simulink model "TxLUT_RxCapture_4x4_HDL_IQ"  (R2019b)
settings: Solver=FixedStepDiscrete  StartTime=0.0  StopTime=15e3  RelTol=1e-3
PreLoadFcn:
  | load('iq_bus_obj.mat');
  | model_init
InitFcn:
  | model_init
values from neighbouring files (symbols this model uses):
  FPGAClkRate = DataSampleRate/VectorSamplingFactor    (= 128000000)    [model_init.m]
  RAM_addr_width = nextpow2(RAM_num_entries)    [model_init.m]
  S2MM_frame_size = 5e4    (= 50000)    [host_io_model_init.m]    (also in model_init.m = length(signal))
  signal = exp(2j*pi*(k/2*t+f0).*t)    [model_init.m]
libraries: hdlsllib x26, simulink x14, rfsoc_hdl_utils x5, dspsrcs4 x2
Description:
  | HDL model for RFSoC ADC/DAC IQ 8x8 interfacing with the mixer enabled
  | 
  | This model contains demonstrates how to interface to all 8 ADC and 8 DAC
  | channels for the RFSoC.
  | 
  | Please ensure that you run the initialization script to set the correct PLL clock rates.
settings Model: DataTypeOverride=Off  SimulationMode=accelerator  Creator=mfornero  LastModifiedBy=ajtro
settings DataIOCC: SaveOutput=off  SaveTime=off  ReturnWorkspaceOutputs=off
settings OptimizationCC: BlockReduction=off  ConditionallyExecuteInputs=off  DefaultParameterBehavior=Inlined  LifeSpan=inf
settings DebuggingCC: AlgebraicLoopMsg=error  SingleTaskRateTransMsg=error  PregeneratedLibrarySubsystemCodeDiagnostic=none  StrictBusMsg=ErrorOnBusTreatedAsVector  SFUnexpectedBacktrackingDiag=warning  SFNoUnconditionalDefaultTransitionDiag=warning  SFExecutionAtInitializationDiag=none  ArithmeticOperatorsInVariantConditions=warning
settings HardwareCC: ProdBitPerPointer=32  ProdBitPerSizeT=32  ProdBitPerPtrDiffT=32  ProdLargestAtomicFloat=None  ProdIntDivRoundTo=Undefined  ProdEndianess=Unspecified  ProdWordSize=32  ProdHWDeviceType=ASIC/FPGA->ASIC/FPGA  ProdEqTarget=off
settings SFSimCC: SimUseLocalCustomCode=off  CustomCodeUndefinedFunction=UseInterfaceOnly
settings RTWCC: RTWUseLocalCustomCode=off
settings CodeAppCC: StateflowObjectComments=on
settings GRTTargetCC: TargetLangStandard=C89/C90 (ANSI)
settings ConfigComp: CovMetricSettings=dw  CovHtmlReporting=on  CovSaveCumulativeToWorkspaceVar=on  CovSaveSingleToWorkspaceVar=on  CovExternalEMLEnable=off

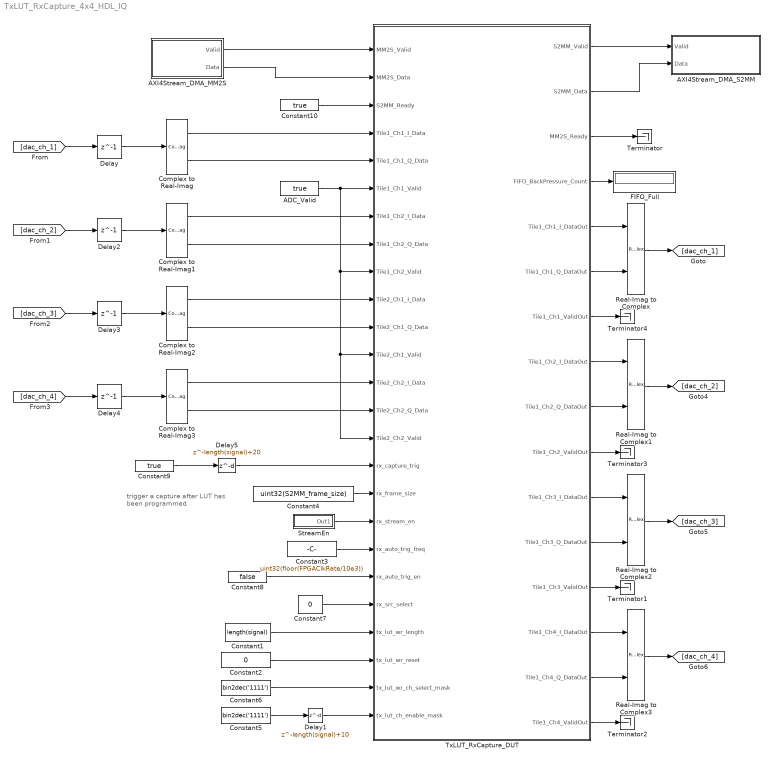
== system TxLUT_RxCapture_4x4_HDL_IQ ==
  note: trigger a capture after LUT
      | has been programmed
  ADC_Valid : Constant  Value=true  SampleTime=-1
  AXI4Stream_DMA_MM2S : Subsystem
  AXI4Stream_DMA_S2MM : Subsystem
  Complex to Real-Imag{,1..3} (4 alike) : ComplexToRealImag
  Constant1 : Constant  Value=length(signal)  OutDataTypeStr=uint32  SampleTime=-1
  Constant10 : Constant  Value=true  SampleTime=-1
  Constant2 : Constant  Value=0  OutDataTypeStr=boolean  SampleTime=-1
  Constant3 : Constant  Value=uint32(floor(FPGAClkRate/10e3))  OutDataTypeStr=uint32  SampleTime=-1
  Constant4 : Constant  Value=uint32(S2MM_frame_size)  SampleTime=-1
  Constant5 : Constant  Value=bin2dec('1111')  OutDataTypeStr=uint32  SampleTime=-1
  Constant6 : Constant  Value=bin2dec('1111')  OutDataTypeStr=uint32  SampleTime=-1
  Constant7 : Constant  Value=0  OutDataTypeStr=fixdt(0,1,0)  SampleTime=-1
  Constant8 : Constant  Value=false  SampleTime=-1
  Constant9 : Constant  Value=true  SampleTime=-1
  Delay{,2..4} (4 alike) : Delay  DelayLength=1
  Delay1 : Delay  DelayLength=length(signal)+10
  Delay5 : Delay  DelayLength=length(signal)+20
  FIFO_Full : Display
  Real-Imag to Complex{,1..3} (4 alike) : RealImagToComplex
  StreamEn : Subsystem
  Terminator{,1..4} (5 alike) : Terminator
  TxLUT_RxCapture_DUT : Subsystem  TreatAsAtomicUnit=on
  wires:
  Constant4/1 -> TxLUT_RxCapture_DUT/17(rx_frame_size)
  StreamEn/1(Out1) -> TxLUT_RxCapture_DUT/18(rx_stream_en)
  Constant3/1 -> TxLUT_RxCapture_DUT/19(rx_auto_trig_freq)
  TxLUT_RxCapture_DUT/1(S2MM_Valid) -> AXI4Stream_DMA_S2MM/1(Valid)
  TxLUT_RxCapture_DUT/2(S2MM_Data) -> AXI4Stream_DMA_S2MM/2(Data)
  TxLUT_RxCapture_DUT/3(MM2S_Ready) -> Terminator/1
  ADC_Valid/1 -> TxLUT_RxCapture_DUT/9(Tile1_Ch2_Valid), TxLUT_RxCapture_DUT/12(Tile2_Ch1_Valid), TxLUT_RxCapture_DUT/15(Tile2_Ch2_Valid), TxLUT_RxCapture_DUT/6(Tile1_Ch1_Valid)
  Constant1/1 -> TxLUT_RxCapture_DUT/22(tx_lut_wr_length)
  AXI4Stream_DMA_MM2S/1(Valid) -> TxLUT_RxCapture_DUT/1(MM2S_Valid)
  AXI4Stream_DMA_MM2S/2(Data) -> TxLUT_RxCapture_DUT/2(MM2S_Data)
  Constant10/1 -> TxLUT_RxCapture_DUT/3(S2MM_Ready)
  Constant2/1 -> TxLUT_RxCapture_DUT/23(tx_lut_wr_reset)
  Constant5/1 -> Delay1/1
  Constant6/1 -> TxLUT_RxCapture_DUT/24(tx_lut_wr_ch_select_mask)
  Complex to Real-Imag/1 -> TxLUT_RxCapture_DUT/4("Tile1_Ch1_I_Data ")
  Delay/1 -> Complex to Real-Imag/1
  Delay1/1 -> TxLUT_RxCapture_DUT/25(tx_lut_ch_enable_mask)
  Complex to Real-Imag/2 -> TxLUT_RxCapture_DUT/5(Tile1_Ch1_Q_Data)
  Constant7/1 -> TxLUT_RxCapture_DUT/21(rx_src_select)
  TxLUT_RxCapture_DUT/5(Tile1_Ch1_I_DataOut) -> Real-Imag to Complex/1
  TxLUT_RxCapture_DUT/6(Tile1_Ch1_Q_DataOut) -> Real-Imag to Complex/2
  TxLUT_RxCapture_DUT/4(FIFO_BackPressure_Count) -> FIFO_Full/1
  TxLUT_RxCapture_DUT/8(Tile1_Ch2_I_DataOut) -> Real-Imag to Complex1/1
  TxLUT_RxCapture_DUT/9(Tile1_Ch2_Q_DataOut) -> Real-Imag to Complex1/2
  TxLUT_RxCapture_DUT/11(Tile1_Ch3_I_DataOut) -> Real-Imag to Complex2/1
  TxLUT_RxCapture_DUT/12(Tile1_Ch3_Q_DataOut) -> Real-Imag to Complex2/2
  TxLUT_RxCapture_DUT/14(Tile1_Ch4_I_DataOut) -> Real-Imag to Complex3/1
  TxLUT_RxCapture_DUT/15(Tile1_Ch4_Q_DataOut) -> Real-Imag to Complex3/2
  TxLUT_RxCapture_DUT/13(Tile1_Ch3_ValidOut) -> Terminator1/1
  TxLUT_RxCapture_DUT/16(Tile1_Ch4_ValidOut) -> Terminator2/1
  TxLUT_RxCapture_DUT/10(Tile1_Ch2_ValidOut) -> Terminator3/1
  TxLUT_RxCapture_DUT/7(Tile1_Ch1_ValidOut) -> Terminator4/1
  Real-Imag to Complex/1 -> [dac_ch_1]
  Real-Imag to Complex1/1 -> [dac_ch_2]
  Real-Imag to Complex2/1 -> [dac_ch_3]
  Real-Imag to Complex3/1 -> [dac_ch_4]
  [dac_ch_1] -> Delay/1
  [dac_ch_2] -> Delay2/1
  Complex to Real-Imag1/2 -> TxLUT_RxCapture_DUT/8(Tile1_Ch2_Q_Data)
  Delay2/1 -> Complex to Real-Imag1/1
  Complex to Real-Imag1/1 -> TxLUT_RxCapture_DUT/7(Tile1_Ch2_I_Data)
  Complex to Real-Imag2/1 -> TxLUT_RxCapture_DUT/10(Tile2_Ch1_I_Data)
  Delay3/1 -> Complex to Real-Imag2/1
  Complex to Real-Imag2/2 -> TxLUT_RxCapture_DUT/11(Tile2_Ch1_Q_Data)
  [dac_ch_3] -> Delay3/1
  [dac_ch_4] -> Delay4/1
  Complex to Real-Imag3/2 -> TxLUT_RxCapture_DUT/14(Tile2_Ch2_Q_Data)
  Delay4/1 -> Complex to Real-Imag3/1
  Complex to Real-Imag3/1 -> TxLUT_RxCapture_DUT/13(Tile2_Ch2_I_Data)
  Constant8/1 -> TxLUT_RxCapture_DUT/20(rx_auto_trig_en)
  Constant9/1 -> Delay5/1
  Delay5/1 -> TxLUT_RxCapture_DUT/16(rx_capture_trig)

== system TxLUT_RxCapture_4x4_HDL_IQ/AXI4Stream_DMA_MM2S ==
  note: Simple behavioral model for MM2S DMA
  Data Type Conversion : DataTypeConversion  OutDataTypeStr=fixdt(0,128,0)  ConvertRealWorld=Stored Integer (SI)
  Pack Complex : rfsoc_hdl_utils/Pack Complex  dummy=0
  Signal From Workspace : dspsrcs4/Signal From Workspace  X=signal_int16  Ts=1  nsamps=1  OutputAfterFinalValue=Setting to zero  ignoreOrWarnInputAndFrameLengths=off  OutputFrames=off
  Signal From Workspace1 : dspsrcs4/Signal From Workspace  X=true(length(signal),1)  Ts=1  nsamps=1  OutputAfterFinalValue=Setting to zero  ignoreOrWarnInputAndFrameLengths=off  OutputFrames=off
  Valid : Outport  VectorParamsAs1DForOutWhenUnconnected=off
  Data : Outport  Port=2  VectorParamsAs1DForOutWhenUnconnected=off
  wires:
  Signal From Workspace/1 -> Pack Complex/1
  Signal From Workspace1/1 -> Valid/1
  Data Type Conversion/1 -> Data/1
  Pack Complex/1 -> Data Type Conversion/1

== system TxLUT_RxCapture_4x4_HDL_IQ/AXI4Stream_DMA_S2MM ==
  Valid : Inport
  Data : Inport  Port=2
  PlotData : Subsystem
  wires:
  Valid/1 -> PlotData/Enable
  Data/1 -> PlotData/1(In1)

== system TxLUT_RxCapture_4x4_HDL_IQ/StreamEn ==
  Data Type Conversion1 : DataTypeConversion  OutDataTypeStr=boolean
  Manual Switch1 : ManualSwitch
  OFF : Constant  Value=0  OutDataTypeStr=boolean  SampleTime=-1
  ON : Constant  OutDataTypeStr=boolean  SampleTime=-1
  Out1 : Outport  VectorParamsAs1DForOutWhenUnconnected=off
  wires:
  Data Type Conversion1/1 -> Out1/1
  OFF/1 -> Manual Switch1/2
  ON/1 -> Manual Switch1/1
  Manual Switch1/1 -> Data Type Conversion1/1

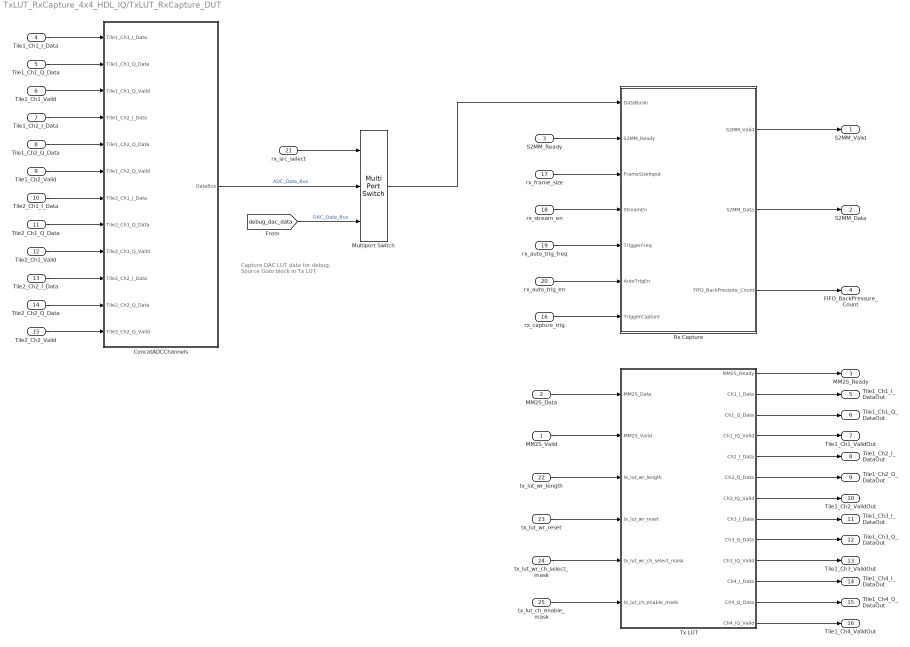
== system TxLUT_RxCapture_4x4_HDL_IQ/TxLUT_RxCapture_DUT ==
  note: Capture DAC LUT data for debug,
      | Source Goto block in Tx LUT
  MM2S_Valid : Inport
  MM2S_Data : Inport  Port=2
  S2MM_Ready : Inport  Port=3
  "Tile1_Ch1_I_Data " : Inport  Port=4
  Tile1_Ch1_Q_Data : Inport  Port=5
  Tile1_Ch1_Valid : Inport  Port=6
  Tile1_Ch2_I_Data : Inport  Port=7
  Tile1_Ch2_Q_Data : Inport  Port=8
  Tile1_Ch2_Valid : Inport  Port=9
  Tile2_Ch1_I_Data : Inport  Port=10
  Tile2_Ch1_Q_Data : Inport  Port=11
  Tile2_Ch1_Valid : Inport  Port=12
  Tile2_Ch2_I_Data : Inport  Port=13
  Tile2_Ch2_Q_Data : Inport  Port=14
  Tile2_Ch2_Valid : Inport  Port=15
  rx_capture_trig : Inport  Port=16
  rx_frame_size : Inport  Port=17
  rx_stream_en : Inport  Port=18
  rx_auto_trig_freq : Inport  Port=19
  rx_auto_trig_en : Inport  Port=20
  rx_src_select : Inport  Port=21  OutDataTypeStr=fixdt(0,1,0)
  tx_lut_wr_length : Inport  Port=22
  tx_lut_wr_reset : Inport  Port=23
  tx_lut_wr_ch_select_mask : Inport  Port=24
  tx_lut_ch_enable_mask : Inport  Port=25
  ConcatADCChannels : Subsystem
  Multiport Switch : MultiPortSwitch  DataPortOrder=Zero-based contiguous  Inputs=2  zeroidx=on
  Rx Capture : Subsystem
  Tx LUT : Subsystem
  S2MM_Valid : Outport  VectorParamsAs1DForOutWhenUnconnected=off
  S2MM_Data : Outport  Port=2  VectorParamsAs1DForOutWhenUnconnected=off
  MM2S_Ready : Outport  Port=3  VectorParamsAs1DForOutWhenUnconnected=off
  FIFO_BackPressure_Count : Outport  Port=4  VectorParamsAs1DForOutWhenUnconnected=off
  Tile1_Ch1_I_DataOut : Outport  Port=5  VectorParamsAs1DForOutWhenUnconnected=off
  Tile1_Ch1_Q_DataOut : Outport  Port=6  VectorParamsAs1DForOutWhenUnconnected=off
  Tile1_Ch1_ValidOut : Outport  Port=7  VectorParamsAs1DForOutWhenUnconnected=off
  Tile1_Ch2_I_DataOut : Outport  Port=8  VectorParamsAs1DForOutWhenUnconnected=off
  Tile1_Ch2_Q_DataOut : Outport  Port=9  VectorParamsAs1DForOutWhenUnconnected=off
  Tile1_Ch2_ValidOut : Outport  Port=10  VectorParamsAs1DForOutWhenUnconnected=off
  Tile1_Ch3_I_DataOut : Outport  Port=11  VectorParamsAs1DForOutWhenUnconnected=off
  Tile1_Ch3_Q_DataOut : Outport  Port=12  VectorParamsAs1DForOutWhenUnconnected=off
  Tile1_Ch3_ValidOut : Outport  Port=13  VectorParamsAs1DForOutWhenUnconnected=off
  Tile1_Ch4_I_DataOut : Outport  Port=14  VectorParamsAs1DForOutWhenUnconnected=off
  Tile1_Ch4_Q_DataOut : Outport  Port=15  VectorParamsAs1DForOutWhenUnconnected=off
  Tile1_Ch4_ValidOut : Outport  Port=16  VectorParamsAs1DForOutWhenUnconnected=off
  wires:
  Tx LUT/1(MM2S_Ready) -> MM2S_Ready/1
  S2MM_Ready/1 -> Rx Capture/2(S2MM_Ready)
  rx_frame_size/1 -> Rx Capture/3(FrameSizeInput)
  rx_stream_en/1 -> Rx Capture/4(StreamEn)
  rx_auto_trig_freq/1 -> Rx Capture/5(TriggerFreq)
  rx_auto_trig_en/1 -> Rx Capture/6(AutoTrigEn)
  rx_capture_trig/1 -> Rx Capture/7(TriggerCapture)
  Rx Capture/1(S2MM_Valid) -> S2MM_Valid/1
  Rx Capture/2(S2MM_Data) -> S2MM_Data/1
  Rx Capture/3(FIFO_BackPressure_Count) -> FIFO_BackPressure_Count/1
  MM2S_Data/1 -> Tx LUT/1(MM2S_Data)
  MM2S_Valid/1 -> Tx LUT/2(MM2S_Valid)
  tx_lut_wr_ch_select_mask/1 -> Tx LUT/5(tx_lut_wr_ch_select_mask)
  tx_lut_wr_length/1 -> Tx LUT/3(tx_lut_wr_length)
  tx_lut_wr_reset/1 -> Tx LUT/4(tx_lut_wr_reset)
  tx_lut_ch_enable_mask/1 -> Tx LUT/6(tx_lut_ch_enable_mask)
  "Tile1_Ch1_I_Data "/1 -> ConcatADCChannels/1("Tile1_Ch1_I_Data ")
  Tile1_Ch1_Q_Data/1 -> ConcatADCChannels/2(Tile1_Ch1_Q_Data)
  Tile1_Ch1_Valid/1 -> ConcatADCChannels/3(Tile1_Ch1_Q_Valid)
  Tile1_Ch2_I_Data/1 -> ConcatADCChannels/4(Tile1_Ch2_I_Data)
  Tile1_Ch2_Q_Data/1 -> ConcatADCChannels/5(Tile1_Ch2_Q_Data)
  Tile1_Ch2_Valid/1 -> ConcatADCChannels/6(Tile1_Ch2_Q_Valid)
  Tile2_Ch1_I_Data/1 -> ConcatADCChannels/7(Tile2_Ch1_I_Data)
  Tile2_Ch1_Q_Data/1 -> ConcatADCChannels/8(Tile2_Ch1_Q_Data)
  Tile2_Ch1_Valid/1 -> ConcatADCChannels/9(Tile2_Ch1_Q_Valid)
  Tile2_Ch2_I_Data/1 -> ConcatADCChannels/10(Tile2_Ch2_I_Data)
  Tile2_Ch2_Q_Data/1 -> ConcatADCChannels/11(Tile2_Ch2_Q_Data)
  Tile2_Ch2_Valid/1 -> ConcatADCChannels/12(Tile2_Ch2_Q_Valid)
  [debug_dac_data] -> Multiport Switch/3  "DAC_Data_Bus"
  ConcatADCChannels/1(DataBus) -> Multiport Switch/2  "ADC_Data_Bus"
  Multiport Switch/1 -> Rx Capture/1(DataBusIn)
  rx_src_select/1 -> Multiport Switch/1
  Tx LUT/2(Ch1_I_Data) -> Tile1_Ch1_I_DataOut/1
  Tx LUT/11(Ch4_I_Data) -> Tile1_Ch4_I_DataOut/1
  Tx LUT/10(Ch3_IQ_Valid) -> Tile1_Ch3_ValidOut/1
  Tx LUT/13(Ch4_IQ_Valid) -> Tile1_Ch4_ValidOut/1
  Tx LUT/5(Ch2_I_Data) -> Tile1_Ch2_I_DataOut/1
  Tx LUT/4(Ch1_IQ_Valid) -> Tile1_Ch1_ValidOut/1
  Tx LUT/12(Ch4_Q_Data) -> Tile1_Ch4_Q_DataOut/1
  Tx LUT/6(Ch2_Q_Data) -> Tile1_Ch2_Q_DataOut/1
  Tx LUT/3(Ch1_Q_Data) -> Tile1_Ch1_Q_DataOut/1
  Tx LUT/9(Ch3_Q_Data) -> Tile1_Ch3_Q_DataOut/1
  Tx LUT/8(Ch3_I_Data) -> Tile1_Ch3_I_DataOut/1
  Tx LUT/7(Ch2_IQ_Valid) -> Tile1_Ch2_ValidOut/1

== system TxLUT_RxCapture_4x4_HDL_IQ/AXI4Stream_DMA_S2MM/PlotData ==
  In1 : Inport
  Enable : EnablePort
  Channel Unpack : rfsoc_hdl_utils/Channel Unpack  samplesPerClock=4  complexSamples=on  reqBitWidth=0
  Demux : Demux
  Spectrum Analyzer : SpectrumAnalyzer
  Time Scope : Scope  NumInputPorts=4
  wires:
  In1/1 -> Channel Unpack/1
  Channel Unpack/1 -> Demux/1
  Demux/2 -> Time Scope/2
  Demux/1 -> Spectrum Analyzer/1, Time Scope/1
  Demux/3 -> Time Scope/3
  Demux/4 -> Time Scope/4

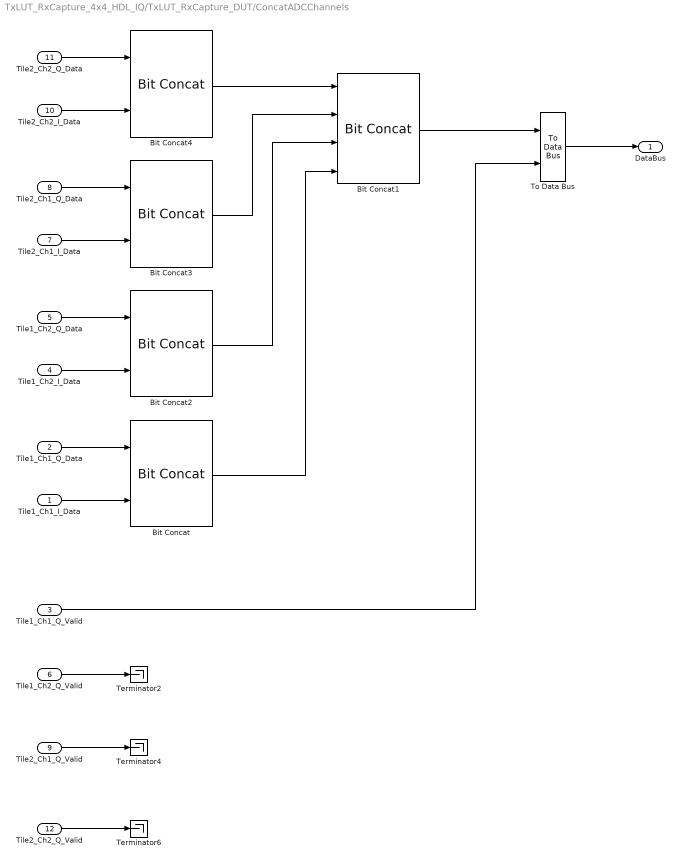
== system TxLUT_RxCapture_4x4_HDL_IQ/TxLUT_RxCapture_DUT/ConcatADCChannels ==
  "Tile1_Ch1_I_Data " : Inport
  Tile1_Ch1_Q_Data : Inport  Port=2
  Tile1_Ch1_Q_Valid : Inport  Port=3
  Tile1_Ch2_I_Data : Inport  Port=4
  Tile1_Ch2_Q_Data : Inport  Port=5
  Tile1_Ch2_Q_Valid : Inport  Port=6
  Tile2_Ch1_I_Data : Inport  Port=7
  Tile2_Ch1_Q_Data : Inport  Port=8
  Tile2_Ch1_Q_Valid : Inport  Port=9
  Tile2_Ch2_I_Data : Inport  Port=10
  Tile2_Ch2_Q_Data : Inport  Port=11
  Tile2_Ch2_Q_Valid : Inport  Port=12
  Bit Concat{,2..4} (4 alike) : hdlsllib/Logic and Bit Operations/Bit Concat  numInputs=2
      settings: SourceProductName=Simulink
  Bit Concat1 : hdlsllib/Logic and Bit Operations/Bit Concat  numInputs=4
      settings: SourceProductName=Simulink
  Terminator2 : Terminator
  Terminator4 : Terminator
  Terminator6 : Terminator
  To Data Bus : rfsoc_hdl_utils/To Data Bus  dummy=0
  DataBus : Outport  VectorParamsAs1DForOutWhenUnconnected=off
  wires:
  Tile1_Ch2_Q_Valid/1 -> Terminator2/1
  Tile1_Ch1_Q_Valid/1 -> To Data Bus/2
  Tile2_Ch2_Q_Valid/1 -> Terminator6/1
  Tile2_Ch1_Q_Valid/1 -> Terminator4/1
  Bit Concat4/1 -> Bit Concat1/1
  Bit Concat3/1 -> Bit Concat1/2
  Bit Concat2/1 -> Bit Concat1/3
  Bit Concat/1 -> Bit Concat1/4
  "Tile1_Ch1_I_Data "/1 -> Bit Concat/2
  Tile1_Ch1_Q_Data/1 -> Bit Concat/1
  Tile1_Ch2_Q_Data/1 -> Bit Concat2/1
  Tile1_Ch2_I_Data/1 -> Bit Concat2/2
  Tile2_Ch1_Q_Data/1 -> Bit Concat3/1
  Tile2_Ch1_I_Data/1 -> Bit Concat3/2
  Tile2_Ch2_Q_Data/1 -> Bit Concat4/1
  Tile2_Ch2_I_Data/1 -> Bit Concat4/2
  Bit Concat1/1 -> To Data Bus/1
  To Data Bus/1 -> DataBus/1

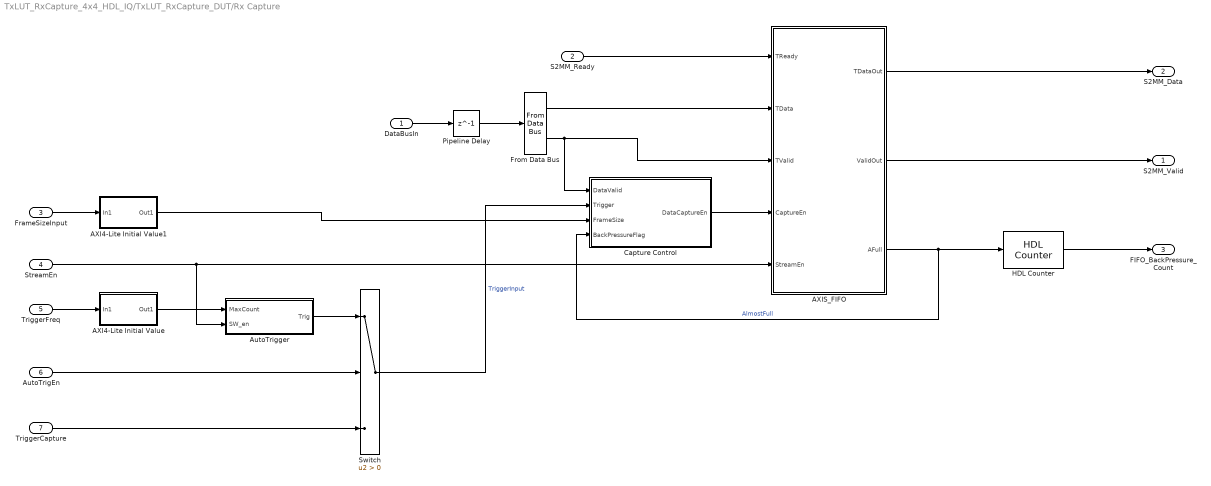
== system TxLUT_RxCapture_4x4_HDL_IQ/TxLUT_RxCapture_DUT/Rx Capture ==
  DataBusIn : Inport
  S2MM_Ready : Inport  Port=2
  FrameSizeInput : Inport  Port=3
  StreamEn : Inport  Port=4
  TriggerFreq : Inport  Port=5
  AutoTrigEn : Inport  Port=6
  TriggerCapture : Inport  Port=7
  " AXIS_FIFO" : Subsystem
  AXI4-Lite Initial Value : Subsystem  mask(AXI4-Lite Initial Value){x0=uint32(floor(FPGAClkRate/2))}
      mask prompts: x0 "Initial value:"
      mask help: Set the initial value for an AXI4-Lite register.
      mask Display: fprintf('x0 = %g',x0);
  AXI4-Lite Initial Value1 : Subsystem  mask(AXI4-Lite Initial Value){x0=16384}
      mask prompts: x0 "Initial value:"
      mask help: Set the initial value for an AXI4-Lite register.
      mask Display: fprintf('x0 = %g',x0);
  AutoTrigger : Subsystem
  Capture Control : Subsystem
  From Data Bus : rfsoc_hdl_utils/From Data Bus  dummy=0
  HDL Counter : hdlsllib/Sources/HDL Counter  CountType=Free running  CountInit=0  CountStep=1  CountMax=25  CountFromType=Initial value  CountFrom=0  CountResetPort=off  CountLoadPort=off  CountEnbPort=on  CountDirPort=off  CountDataType=Unsigned  CountWordLen=32  CountFracLen=0  CountSampTime=1
      settings: SourceProductName=Simulink
  Pipeline Delay : Delay  DelayLength=1  InitialCondition=0
  Switch : Switch  Criteria=u2 > Threshold
  S2MM_Valid : Outport  VectorParamsAs1DForOutWhenUnconnected=off
  S2MM_Data : Outport  Port=2  VectorParamsAs1DForOutWhenUnconnected=off
  FIFO_BackPressure_Count : Outport  Port=3  VectorParamsAs1DForOutWhenUnconnected=off
  wires:
  StreamEn/1 -> AutoTrigger/2(SW_en), " AXIS_FIFO"/5(StreamEn)
  From Data Bus/2 -> Capture Control/1(DataValid), " AXIS_FIFO"/3(TValid)
  AutoTrigger/1(Trig) -> Switch/1
  FrameSizeInput/1 -> AXI4-Lite Initial Value1/1(In1)
  S2MM_Ready/1 -> " AXIS_FIFO"/1(TReady)
  TriggerCapture/1 -> Switch/3
  " AXIS_FIFO"/3(AFull) -> Capture Control/4(BackPressureFlag), HDL Counter/1  "AlmostFull"
  " AXIS_FIFO"/2(ValidOut) -> S2MM_Valid/1
  Capture Control/1(DataCaptureEn) -> " AXIS_FIFO"/4(CaptureEn)
  TriggerFreq/1 -> AXI4-Lite Initial Value/1(In1)
  AXI4-Lite Initial Value/1(Out1) -> AutoTrigger/1(MaxCount)
  AutoTrigEn/1 -> Switch/2
  From Data Bus/1 -> " AXIS_FIFO"/2(TData)
  Switch/1 -> Capture Control/2(Trigger)  "TriggerInput"
  HDL Counter/1 -> FIFO_BackPressure_Count/1
  " AXIS_FIFO"/1(TDataOut) -> S2MM_Data/1
  DataBusIn/1 -> Pipeline Delay/1
  AXI4-Lite Initial Value1/1(Out1) -> Capture Control/3(FrameSize)
  Pipeline Delay/1 -> From Data Bus/1

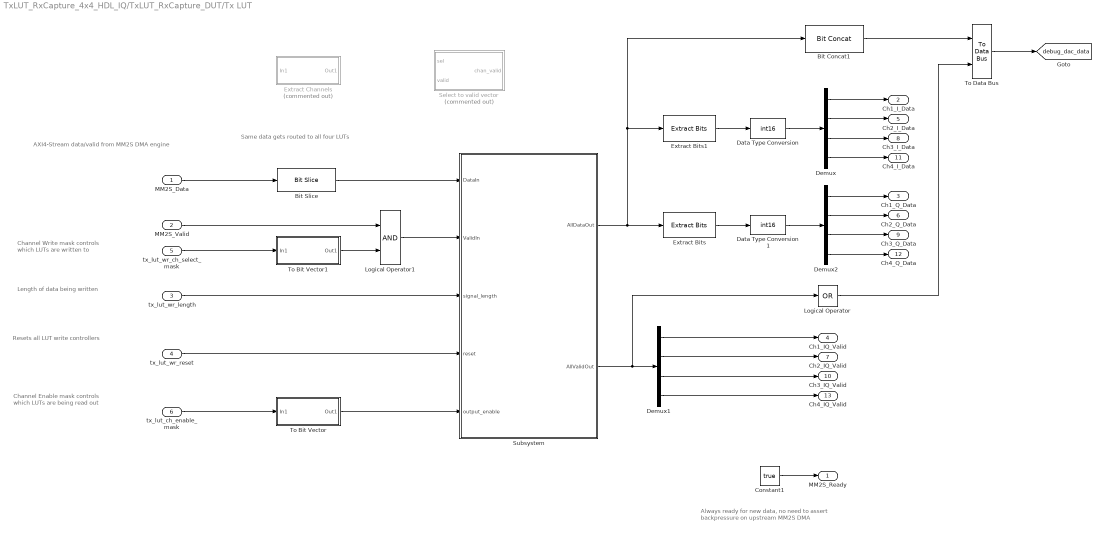
== system TxLUT_RxCapture_4x4_HDL_IQ/TxLUT_RxCapture_DUT/Tx LUT ==
  note: AXI4-Stream data/valid from MM2S DMA engine
  note: Always ready for new data, no need to assert
      | backpressure on upstream MM2S DMA
  note: Length of data being written
  note: Resets all LUT write controllers
  note: Channel Enable mask controls
      | which LUTs are being read out
  note: Channel Write mask controls
      | which LUTs are written to
  note: Same data gets routed to all four LUTs
  MM2S_Data : Inport
  MM2S_Valid : Inport  Port=2
  tx_lut_wr_length : Inport  Port=3
  tx_lut_wr_reset : Inport  Port=4
  tx_lut_wr_ch_select_mask : Inport  Port=5
  tx_lut_ch_enable_mask : Inport  Port=6
  Bit Concat1 : hdlsllib/Logic and Bit Operations/Bit Concat  numInputs=1
      settings: SourceProductName=Simulink
  Bit Slice : hdlsllib/Logic and Bit Operations/Bit Slice  lidx=31  ridx=0
      settings: SourceProductName=Simulink  SourceProductBaseCode=SL
  Constant1 : Constant  Value=true  OutDataTypeStr=boolean  SampleTime=-1
  Data Type Conversion : DataTypeConversion  OutDataTypeStr=int16  ConvertRealWorld=Stored Integer (SI)
  Data Type Conversion1 : DataTypeConversion  OutDataTypeStr=int16  ConvertRealWorld=Stored Integer (SI)
  Demux : Demux  Outputs=NumChan
  Demux1 : Demux  Outputs=NumChan
  Demux2 : Demux  Outputs=NumChan
  Extract Bits : simulink/Logic and Bit Operations/Extract Bits  bitsToExtract=Upper half  numBits=8  bitIdxRange=[0 7]  outScalingMode=Treat bit field as an integer
      settings: SourceProductName=Simulink
  Extract Bits1 : simulink/Logic and Bit Operations/Extract Bits  bitsToExtract=Lower half  numBits=8  bitIdxRange=[0 7]  outScalingMode=Treat bit field as an integer
      settings: SourceProductName=Simulink
  Extract Channels : Subsystem  Commented=on
  Logical Operator : Logic  Operator=OR  Inputs=1  IconShape=distinctive  AllPortsSameDT=off  OutDataTypeStr=boolean
  Logical Operator1 : Logic  IconShape=distinctive  AllPortsSameDT=off  OutDataTypeStr=boolean
  Select to valid vector : Subsystem  Commented=on
  Subsystem : Subsystem
  To Bit Vector : Subsystem
  To Bit Vector1 : Subsystem
  To Data Bus : rfsoc_hdl_utils/To Data Bus  dummy=0
  MM2S_Ready : Outport  VectorParamsAs1DForOutWhenUnconnected=off
  Ch1_I_Data : Outport  Port=2  VectorParamsAs1DForOutWhenUnconnected=off
  Ch1_Q_Data : Outport  Port=3  VectorParamsAs1DForOutWhenUnconnected=off
  Ch1_IQ_Valid : Outport  Port=4  VectorParamsAs1DForOutWhenUnconnected=off
  Ch2_I_Data : Outport  Port=5  VectorParamsAs1DForOutWhenUnconnected=off
  Ch2_Q_Data : Outport  Port=6  VectorParamsAs1DForOutWhenUnconnected=off
  Ch2_IQ_Valid : Outport  Port=7  VectorParamsAs1DForOutWhenUnconnected=off
  Ch3_I_Data : Outport  Port=8  VectorParamsAs1DForOutWhenUnconnected=off
  Ch3_Q_Data : Outport  Port=9  VectorParamsAs1DForOutWhenUnconnected=off
  Ch3_IQ_Valid : Outport  Port=10  VectorParamsAs1DForOutWhenUnconnected=off
  Ch4_I_Data : Outport  Port=11  VectorParamsAs1DForOutWhenUnconnected=off
  Ch4_Q_Data : Outport  Port=12  VectorParamsAs1DForOutWhenUnconnected=off
  Ch4_IQ_Valid : Outport  Port=13  VectorParamsAs1DForOutWhenUnconnected=off
  tag scope: debug_dac_data=global
  wires:
  tx_lut_ch_enable_mask/1 -> To Bit Vector/1(In1)
  tx_lut_wr_length/1 -> Subsystem/3(signal_length)
  MM2S_Data/1 -> Bit Slice/1
  tx_lut_wr_ch_select_mask/1 -> To Bit Vector1/1(In1)
  Subsystem/1(AllDataOut) -> Extract Bits/1, Bit Concat1/1, Extract Bits1/1
  Subsystem/2(AllValidOut) -> Logical Operator/1, Demux1/1
  Demux/1 -> Ch1_I_Data/1
  Demux1/1 -> Ch1_IQ_Valid/1
  Demux/2 -> Ch2_I_Data/1
  Demux1/2 -> Ch2_IQ_Valid/1
  Demux/3 -> Ch3_I_Data/1
  Demux1/3 -> Ch3_IQ_Valid/1
  Demux/4 -> Ch4_I_Data/1
  Demux1/4 -> Ch4_IQ_Valid/1
  To Bit Vector/1(Out1) -> Subsystem/5(output_enable)
  Bit Slice/1 -> Subsystem/1(DataIn)
  Bit Concat1/1 -> To Data Bus/1
  To Data Bus/1 -> [debug_dac_data]
  Logical Operator/1 -> To Data Bus/2
  Logical Operator1/1 -> Subsystem/2(ValidIn)
  Demux2/4 -> Ch4_Q_Data/1
  Demux2/3 -> Ch3_Q_Data/1
  Demux2/2 -> Ch2_Q_Data/1
  Demux2/1 -> Ch1_Q_Data/1
  Extract Bits/1 -> Data Type Conversion1/1
  Extract Bits1/1 -> Data Type Conversion/1
  Data Type Conversion/1 -> Demux/1
  Data Type Conversion1/1 -> Demux2/1
  tx_lut_wr_reset/1 -> Subsystem/4(reset)
  Constant1/1 -> MM2S_Ready/1
  To Bit Vector1/1(Out1) -> Logical Operator1/2
  MM2S_Valid/1 -> Logical Operator1/1

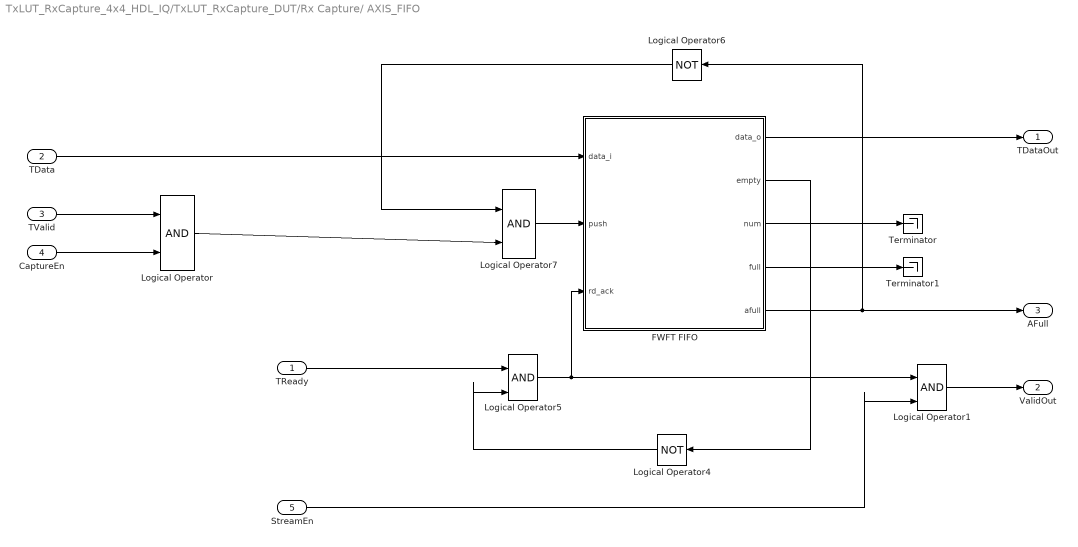
== system TxLUT_RxCapture_4x4_HDL_IQ/TxLUT_RxCapture_DUT/Rx Capture/ AXIS_FIFO ==
  TReady : Inport
  TData : Inport  Port=2
  TValid : Inport  Port=3
  CaptureEn : Inport  Port=4
  StreamEn : Inport  Port=5
  FWFT FIFO : Subsystem  mask{FIFO_DEPTH=1024*10, AFULL_THRESH=10}
      mask prompts: FIFO_DEPTH "FIFO Depth"; AFULL_THRESH "Almost Full Threshold"
      mask init:
      | FIFO_CNT_BITS=ceil(log2(FIFO_DEPTH+1+3));
  Logical Operator{,1,5,7} (4 alike) : Logic  IconShape=distinctive  AllPortsSameDT=off  OutDataTypeStr=boolean
  Logical Operator4 : Logic  Operator=NOT  IconShape=distinctive  AllPortsSameDT=off  OutDataTypeStr=boolean
  Logical Operator6 : Logic  Operator=NOT  IconShape=distinctive  AllPortsSameDT=off  OutDataTypeStr=boolean
  Terminator : Terminator
  Terminator1 : Terminator
  TDataOut : Outport  VectorParamsAs1DForOutWhenUnconnected=off
  ValidOut : Outport  Port=2  VectorParamsAs1DForOutWhenUnconnected=off
  AFull : Outport  Port=3  VectorParamsAs1DForOutWhenUnconnected=off
  wires:
  TValid/1 -> Logical Operator/1
  Logical Operator6/1 -> Logical Operator7/1
  Logical Operator4/1 -> Logical Operator5/2
  Logical Operator5/1 -> Logical Operator1/1, FWFT FIFO/3(rd_ack)
  Logical Operator7/1 -> FWFT FIFO/2(push)
  TReady/1 -> Logical Operator5/1
  FWFT FIFO/5(afull) -> AFull/1, Logical Operator6/1
  Logical Operator/1 -> Logical Operator7/2
  FWFT FIFO/2(empty) -> Logical Operator4/1
  CaptureEn/1 -> Logical Operator/2
  TData/1 -> FWFT FIFO/1(data_i)
  FWFT FIFO/1(data_o) -> TDataOut/1
  Logical Operator1/1 -> ValidOut/1
  StreamEn/1 -> Logical Operator1/2
  FWFT FIFO/3(num) -> Terminator/1
  FWFT FIFO/4(full) -> Terminator1/1

== system TxLUT_RxCapture_4x4_HDL_IQ/TxLUT_RxCapture_DUT/Rx Capture/AXI4-Lite Initial Value ==
  In1 : Inport
  Compare To Zero : simulink/Logic and Bit Operations/Compare To Zero  relop=~=  OutDataTypeStr=boolean
  Logical Operator : Logic  Operator=OR  IconShape=distinctive  AllPortsSameDT=off  OutDataTypeStr=boolean
  Set_Latch : Subsystem
  Unit Delay Enabled Synchronous : hdlsllib/Discrete/Unit Delay Enabled Synchronous  InitialCondition=x0  SampleTime=-1
      settings: SourceProductName=HDL Coder  SourceProductBaseCode=HD
  Out1 : Outport  VectorParamsAs1DForOutWhenUnconnected=off
  wires:
  In1/1 -> Unit Delay Enabled Synchronous/1, Compare To Zero/1
  Logical Operator/1 -> Unit Delay Enabled Synchronous/2
  Compare To Zero/1 -> Logical Operator/1, Set_Latch/1(S)
  Set_Latch/1(Q) -> Logical Operator/2
  Unit Delay Enabled Synchronous/1 -> Out1/1

== system TxLUT_RxCapture_4x4_HDL_IQ/TxLUT_RxCapture_DUT/Rx Capture/AXI4-Lite Initial Value1 ==
  In1 : Inport
  Compare To Zero : simulink/Logic and Bit Operations/Compare To Zero  relop=~=  OutDataTypeStr=boolean
  Logical Operator : Logic  Operator=OR  IconShape=distinctive  AllPortsSameDT=off  OutDataTypeStr=boolean
  Set_Latch : Subsystem
  Unit Delay Enabled Synchronous : hdlsllib/Discrete/Unit Delay Enabled Synchronous  InitialCondition=x0  SampleTime=-1
      settings: SourceProductName=HDL Coder  SourceProductBaseCode=HD
  Out1 : Outport  VectorParamsAs1DForOutWhenUnconnected=off
  wires:
  Unit Delay Enabled Synchronous/1 -> Out1/1
  Set_Latch/1(Q) -> Logical Operator/2
  Compare To Zero/1 -> Set_Latch/1(S), Logical Operator/1
  Logical Operator/1 -> Unit Delay Enabled Synchronous/2
  In1/1 -> Compare To Zero/1, Unit Delay Enabled Synchronous/1

== system TxLUT_RxCapture_4x4_HDL_IQ/TxLUT_RxCapture_DUT/Rx Capture/AutoTrigger ==
  MaxCount : Inport
  SW_en : Inport  Port=2
  DataPushFrequency : hdlsllib/Sources/HDL Counter  CountType=Free running  CountInit=0  CountStep=1  CountMax=25  CountFromType=Initial value  CountFrom=0  CountResetPort=on  CountLoadPort=off  CountEnbPort=on  CountDirPort=off  CountDataType=Unsigned  CountWordLen=32  CountFracLen=0  CountSampTime=1
      settings: SourceProductBaseCode=HD
  Detect Increase : simulink/Logic and Bit Operations/Detect Increase  vinit=0.0  OutDataTypeStr=boolean
  Relational Operator : RelationalOperator  Operator===  OutDataTypeStr=boolean  RndMeth=Simplest
  Trig : Outport  VectorParamsAs1DForOutWhenUnconnected=off
  wires:
  Relational Operator/1 -> Detect Increase/1, DataPushFrequency/1
  DataPushFrequency/1 -> Relational Operator/2  "DataPushFrequencyCount"
  Detect Increase/1 -> Trig/1
  SW_en/1 -> DataPushFrequency/2
  MaxCount/1 -> Relational Operator/1

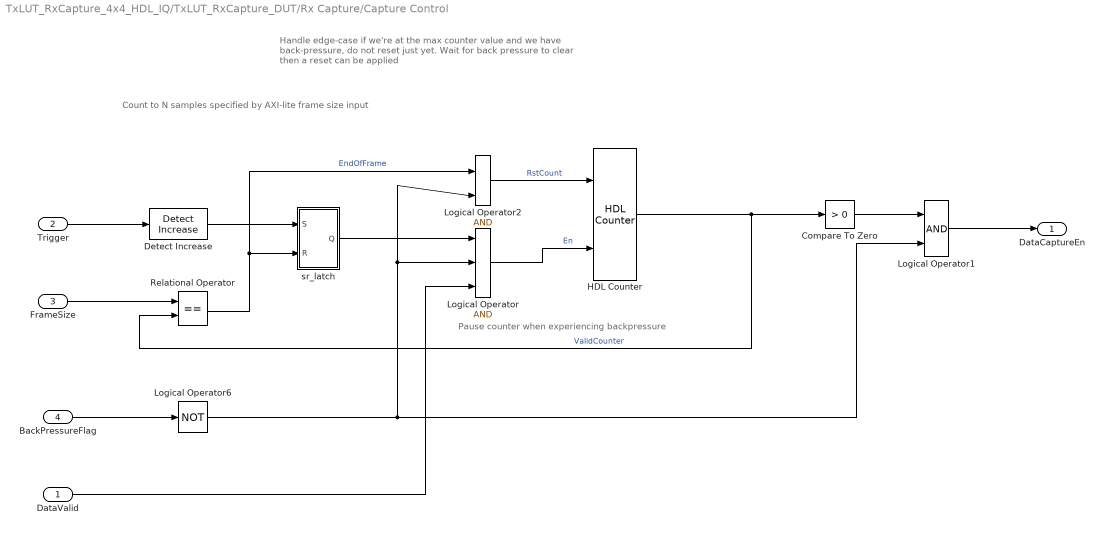
== system TxLUT_RxCapture_4x4_HDL_IQ/TxLUT_RxCapture_DUT/Rx Capture/Capture Control ==
  note: Pause counter when experiencing backpressure
  note: Handle edge-case if we're at the
      | max counter value and we have back-pressure, do not reset
      | just yet. Wait for back pressure to clear then a reset can be applied
  note: Count to N samples specified by AXI-lite frame size input
  DataValid : Inport
  Trigger : Inport  Port=2
  FrameSize : Inport  Port=3
  BackPressureFlag : Inport  Port=4
  Compare To Zero : simulink/Logic and Bit Operations/Compare To Zero  relop=>  OutDataTypeStr=boolean
  Detect Increase : simulink/Logic and Bit Operations/Detect Increase  vinit=0.0  OutDataTypeStr=boolean
  HDL Counter : hdlsllib/Sources/HDL Counter  CountType=Free running  CountInit=0  CountStep=1  CountMax=25  CountFromType=Initial value  CountFrom=0  CountResetPort=on  CountLoadPort=off  CountEnbPort=on  CountDirPort=off  CountDataType=Unsigned  CountWordLen=32  CountFracLen=0  CountSampTime=1
      settings: SourceProductBaseCode=HD
  Logical Operator : Logic  Inputs=3  IconShape=distinctive  AllPortsSameDT=off  OutDataTypeStr=boolean
  Logical Operator1 : Logic  IconShape=distinctive  AllPortsSameDT=off  OutDataTypeStr=boolean
  Logical Operator2 : Logic  IconShape=distinctive  AllPortsSameDT=off  OutDataTypeStr=boolean
  Logical Operator6 : Logic  Operator=NOT  IconShape=distinctive  AllPortsSameDT=off  OutDataTypeStr=boolean
  Relational Operator : RelationalOperator  Operator===  OutDataTypeStr=boolean  RndMeth=Simplest
  sr_latch : Subsystem
  DataCaptureEn : Outport  VectorParamsAs1DForOutWhenUnconnected=off
  wires:
  Logical Operator1/1 -> DataCaptureEn/1
  Detect Increase/1 -> sr_latch/1(S)
  sr_latch/1(Q) -> Logical Operator/1
  HDL Counter/1 -> Compare To Zero/1, Relational Operator/2  "ValidCounter"
  Trigger/1 -> Detect Increase/1
  Logical Operator/1 -> HDL Counter/2  "En"
  Compare To Zero/1 -> Logical Operator1/1
  Relational Operator/1 -> Logical Operator2/1, sr_latch/2(R)  "EndOfFrame"
  BackPressureFlag/1 -> Logical Operator6/1
  Logical Operator2/1 -> HDL Counter/1  "RstCount"
  FrameSize/1 -> Relational Operator/1
  Logical Operator6/1 -> Logical Operator2/2, Logical Operator/2, Logical Operator1/2
  DataValid/1 -> Logical Operator/3

== system TxLUT_RxCapture_4x4_HDL_IQ/TxLUT_RxCapture_DUT/Tx LUT/Extract Channels ==
  In1 : Inport
  Bit Slice : hdlsllib/Logic and Bit Operations/Bit Slice  lidx=31  ridx=0
      settings: SourceProductName=Simulink  SourceProductBaseCode=SL
  Bit Slice1 : hdlsllib/Logic and Bit Operations/Bit Slice  lidx=63  ridx=32
      settings: SourceProductName=Simulink  SourceProductBaseCode=SL
  Bit Slice2 : hdlsllib/Logic and Bit Operations/Bit Slice  lidx=95  ridx=64
      settings: SourceProductName=Simulink  SourceProductBaseCode=SL
  Bit Slice3 : hdlsllib/Logic and Bit Operations/Bit Slice  lidx=127  ridx=96
      settings: SourceProductName=Simulink  SourceProductBaseCode=SL
  Mux : Mux
  Reshape : Reshape  OutputDimensionality=Column vector (2-D)
  Out1 : Outport  VectorParamsAs1DForOutWhenUnconnected=off
  wires:
  Bit Slice1/1 -> Mux/2
  In1/1 -> Bit Slice3/1, Bit Slice2/1, Bit Slice1/1, Bit Slice/1
  Bit Slice2/1 -> Mux/3
  Bit Slice3/1 -> Mux/4
  Bit Slice/1 -> Mux/1
  Reshape/1 -> Out1/1
  Mux/1 -> Reshape/1

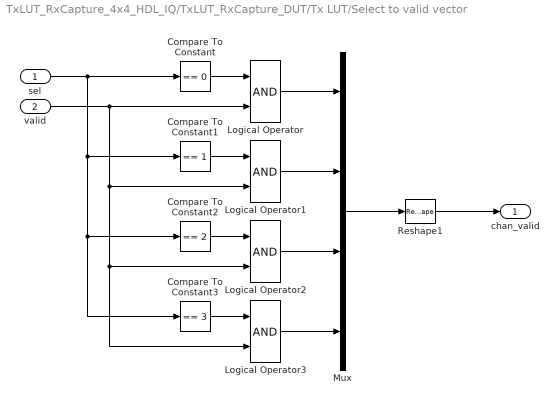
== system TxLUT_RxCapture_4x4_HDL_IQ/TxLUT_RxCapture_DUT/Tx LUT/Select to valid vector ==
  sel : Inport
  valid : Inport  Port=2
  Compare To Constant : simulink/Logic and Bit Operations/Compare To Constant  relop===  const=0  OutDataTypeStr=boolean
  Compare To Constant1 : simulink/Logic and Bit Operations/Compare To Constant  relop===  const=1  OutDataTypeStr=boolean
  Compare To Constant2 : simulink/Logic and Bit Operations/Compare To Constant  relop===  const=2  OutDataTypeStr=boolean
  Compare To Constant3 : simulink/Logic and Bit Operations/Compare To Constant  relop===  const=3  OutDataTypeStr=boolean
  Logical Operator{,1..3} (4 alike) : Logic  IconShape=distinctive  AllPortsSameDT=off  OutDataTypeStr=boolean
  Mux : Mux
  Reshape1 : Reshape  OutputDimensionality=Column vector (2-D)
  chan_valid : Outport  VectorParamsAs1DForOutWhenUnconnected=off
  wires:
  sel/1 -> Compare To Constant1/1, Compare To Constant2/1, Compare To Constant3/1, Compare To Constant/1
  Compare To Constant/1 -> Logical Operator/1
  valid/1 -> Logical Operator1/2, Logical Operator2/2, Logical Operator3/2, Logical Operator/2
  Logical Operator/1 -> Mux/1
  Compare To Constant1/1 -> Logical Operator1/1
  Logical Operator1/1 -> Mux/2
  Compare To Constant2/1 -> Logical Operator2/1
  Logical Operator2/1 -> Mux/3
  Compare To Constant3/1 -> Logical Operator3/1
  Logical Operator3/1 -> Mux/4
  Mux/1 -> Reshape1/1
  Reshape1/1 -> chan_valid/1

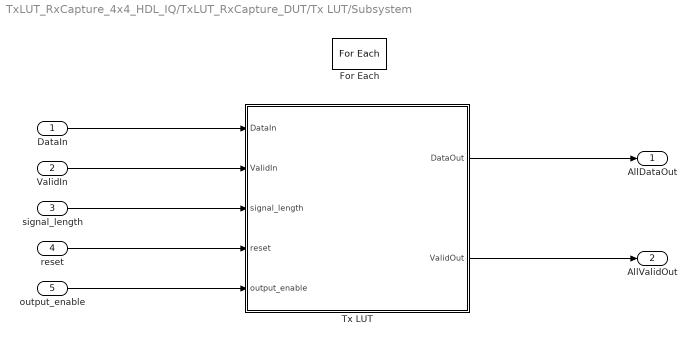
== system TxLUT_RxCapture_4x4_HDL_IQ/TxLUT_RxCapture_DUT/Tx LUT/Subsystem ==
  DataIn : Inport
  ValidIn : Inport  Port=2  Partition=on  PartitionDimension=1  PartitionWidth=1  PartitionOffset=0
  signal_length : Inport  Port=3
  reset : Inport  Port=4
  output_enable : Inport  Port=5  Partition=on  PartitionDimension=1  PartitionWidth=1  PartitionOffset=0
  For Each : ForEach  DisableCoverage=on
  Tx LUT : Subsystem  TreatAsAtomicUnit=on
  AllDataOut : Outport  ConcatenationDimension=1  VectorParamsAs1DForOutWhenUnconnected=off
  AllValidOut : Outport  Port=2  ConcatenationDimension=1  VectorParamsAs1DForOutWhenUnconnected=off
  wires:
  reset/1 -> Tx LUT/4(reset)
  signal_length/1 -> Tx LUT/3(signal_length)
  DataIn/1 -> Tx LUT/1(DataIn)
  ValidIn/1 -> Tx LUT/2(ValidIn)
  Tx LUT/1(DataOut) -> AllDataOut/1
  output_enable/1 -> Tx LUT/5(output_enable)
  Tx LUT/2(ValidOut) -> AllValidOut/1

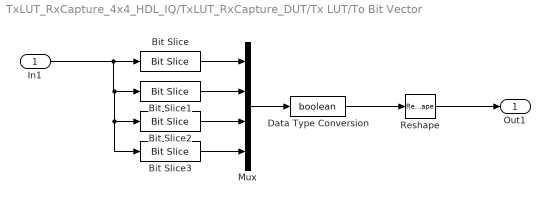
== system TxLUT_RxCapture_4x4_HDL_IQ/TxLUT_RxCapture_DUT/Tx LUT/To Bit Vector ==
  In1 : Inport
  Bit Slice : hdlsllib/Logic and Bit Operations/Bit Slice  lidx=0  ridx=0
      settings: SourceProductName=Simulink  SourceProductBaseCode=SL
  Bit Slice1 : hdlsllib/Logic and Bit Operations/Bit Slice  lidx=1  ridx=1
      settings: SourceProductName=Simulink  SourceProductBaseCode=SL
  Bit Slice2 : hdlsllib/Logic and Bit Operations/Bit Slice  lidx=2  ridx=2
      settings: SourceProductName=Simulink  SourceProductBaseCode=SL
  Bit Slice3 : hdlsllib/Logic and Bit Operations/Bit Slice  lidx=3  ridx=3
      settings: SourceProductName=Simulink  SourceProductBaseCode=SL
  Data Type Conversion : DataTypeConversion  OutDataTypeStr=boolean
  Mux : Mux
  Reshape : Reshape  OutputDimensionality=Column vector (2-D)
  Out1 : Outport  VectorParamsAs1DForOutWhenUnconnected=off
  wires:
  Bit Slice1/1 -> Mux/2
  In1/1 -> Bit Slice3/1, Bit Slice2/1, Bit Slice1/1, Bit Slice/1
  Bit Slice2/1 -> Mux/3
  Bit Slice3/1 -> Mux/4
  Bit Slice/1 -> Mux/1
  Mux/1 -> Data Type Conversion/1
  Reshape/1 -> Out1/1
  Data Type Conversion/1 -> Reshape/1

== system TxLUT_RxCapture_4x4_HDL_IQ/TxLUT_RxCapture_DUT/Tx LUT/To Bit Vector1 ==
  In1 : Inport
  Bit Slice : hdlsllib/Logic and Bit Operations/Bit Slice  lidx=0  ridx=0
      settings: SourceProductName=Simulink  SourceProductBaseCode=SL
  Bit Slice1 : hdlsllib/Logic and Bit Operations/Bit Slice  lidx=1  ridx=1
      settings: SourceProductName=Simulink  SourceProductBaseCode=SL
  Bit Slice2 : hdlsllib/Logic and Bit Operations/Bit Slice  lidx=2  ridx=2
      settings: SourceProductName=Simulink  SourceProductBaseCode=SL
  Bit Slice3 : hdlsllib/Logic and Bit Operations/Bit Slice  lidx=3  ridx=3
      settings: SourceProductName=Simulink  SourceProductBaseCode=SL
  Data Type Conversion : DataTypeConversion  OutDataTypeStr=boolean
  Mux : Mux
  Reshape : Reshape  OutputDimensionality=Column vector (2-D)
  Out1 : Outport  VectorParamsAs1DForOutWhenUnconnected=off
  wires:
  Data Type Conversion/1 -> Reshape/1
  Reshape/1 -> Out1/1
  Mux/1 -> Data Type Conversion/1
  Bit Slice/1 -> Mux/1
  Bit Slice3/1 -> Mux/4
  Bit Slice2/1 -> Mux/3
  In1/1 -> Bit Slice/1, Bit Slice1/1, Bit Slice2/1, Bit Slice3/1
  Bit Slice1/1 -> Mux/2

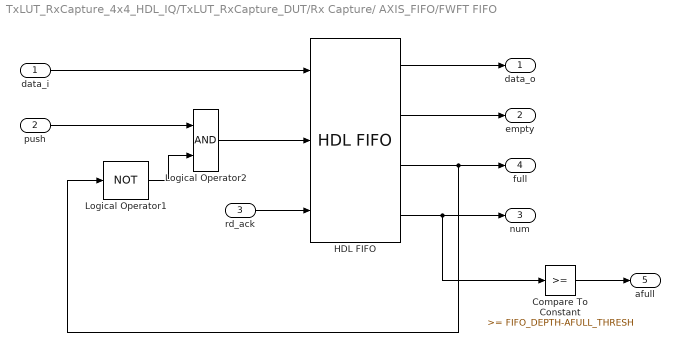
== system TxLUT_RxCapture_4x4_HDL_IQ/TxLUT_RxCapture_DUT/Rx Capture/ AXIS_FIFO/FWFT FIFO ==
  data_i : Inport
  push : Inport  Port=2
  rd_ack : Inport  Port=3
  Compare To Constant : simulink/Logic and Bit Operations/Compare To Constant  relop=>=  const=FIFO_DEPTH-AFULL_THRESH  OutDataTypeStr=boolean
  HDL FIFO : hdlsllib/HDL RAMs/HDL FIFO  fifo_size=FIFO_DEPTH  mode=FWFT  ratio=1  push_msg=Error  pop_msg=Ignore  show_empty=on  show_full=on  show_num=on  LabelModeActiveChoice_Mode=FWFT
      settings: SourceProductName=HDL Coder  SourceProductBaseCode=HD
  Logical Operator1 : Logic  Operator=NOT  IconShape=distinctive  AllPortsSameDT=off  OutDataTypeStr=boolean
  Logical Operator2 : Logic  IconShape=distinctive  AllPortsSameDT=off  OutDataTypeStr=boolean
  data_o : Outport  VectorParamsAs1DForOutWhenUnconnected=off
  empty : Outport  Port=2  VectorParamsAs1DForOutWhenUnconnected=off
  num : Outport  Port=3  VectorParamsAs1DForOutWhenUnconnected=off
  full : Outport  Port=4  VectorParamsAs1DForOutWhenUnconnected=off
  afull : Outport  Port=5  VectorParamsAs1DForOutWhenUnconnected=off
  wires:
  Compare To Constant/1 -> afull/1
  data_i/1 -> HDL FIFO/1
  push/1 -> Logical Operator2/1
  Logical Operator2/1 -> HDL FIFO/2
  Logical Operator1/1 -> Logical Operator2/2
  HDL FIFO/3 -> Logical Operator1/1, full/1
  HDL FIFO/4 -> num/1, Compare To Constant/1
  rd_ack/1 -> HDL FIFO/3
  HDL FIFO/1 -> data_o/1
  HDL FIFO/2 -> empty/1

== system TxLUT_RxCapture_4x4_HDL_IQ/TxLUT_RxCapture_DUT/Rx Capture/AXI4-Lite Initial Value/Set_Latch ==
  S : Inport
  Logical Operator5 : Logic  Operator=OR  IconShape=distinctive  AllPortsSameDT=off  OutDataTypeStr=boolean
  Unit Delay : UnitDelay  SampleTime=-1  HasFrameUpgradeWarning=on
  Q : Outport  VectorParamsAs1DForOutWhenUnconnected=off
  wires:
  Logical Operator5/1 -> Unit Delay/1
  S/1 -> Logical Operator5/1
  Unit Delay/1 -> Q/1, Logical Operator5/2

== system TxLUT_RxCapture_4x4_HDL_IQ/TxLUT_RxCapture_DUT/Rx Capture/AXI4-Lite Initial Value1/Set_Latch ==
  S : Inport
  Logical Operator5 : Logic  Operator=OR  IconShape=distinctive  AllPortsSameDT=off  OutDataTypeStr=boolean
  Unit Delay : UnitDelay  SampleTime=-1  HasFrameUpgradeWarning=on
  Q : Outport  VectorParamsAs1DForOutWhenUnconnected=off
  wires:
  Unit Delay/1 -> Logical Operator5/2, Q/1
  S/1 -> Logical Operator5/1
  Logical Operator5/1 -> Unit Delay/1

== system TxLUT_RxCapture_4x4_HDL_IQ/TxLUT_RxCapture_DUT/Rx Capture/Capture Control/sr_latch ==
  S : Inport
  R : Inport  Port=2
  Logical Operator1 : Logic  IconShape=distinctive  AllPortsSameDT=off  OutDataTypeStr=boolean
  Logical Operator2 : Logic  Operator=NOT  IconShape=distinctive  AllPortsSameDT=off  OutDataTypeStr=boolean
  Logical Operator9 : Logic  Operator=OR  IconShape=distinctive  AllPortsSameDT=off  OutDataTypeStr=boolean
  Unit Delay1 : UnitDelay  SampleTime=-1  HasFrameUpgradeWarning=on
  Q : Outport  VectorParamsAs1DForOutWhenUnconnected=off
  wires:
  S/1 -> Logical Operator9/1
  R/1 -> Logical Operator2/1
  Logical Operator2/1 -> Logical Operator1/1
  Unit Delay1/1 -> Logical Operator1/2, Q/1
  Logical Operator9/1 -> Unit Delay1/1
  Logical Operator1/1 -> Logical Operator9/2

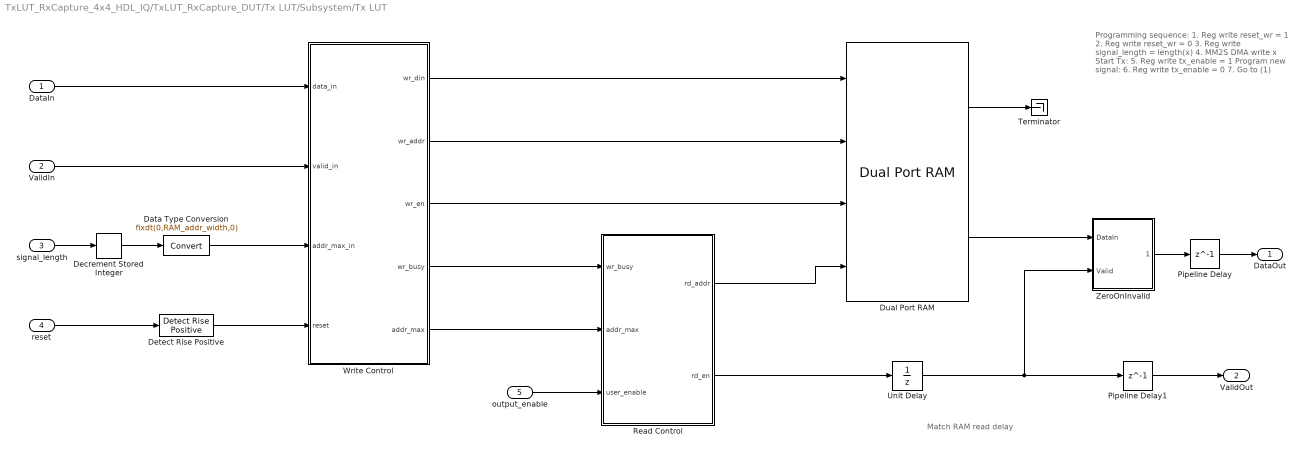
== system TxLUT_RxCapture_4x4_HDL_IQ/TxLUT_RxCapture_DUT/Tx LUT/Subsystem/Tx LUT ==
  note: Match RAM read delay
  note: Programming sequence:
      |
      | 1. Reg write reset_wr = 1
      | 2. Reg write reset_wr = 0
      | 3. Reg write signal_length = length(x)
      | 4. MM2S DMA write x
      |
      | Start Tx:
      | 5. Reg write tx_enable = 1
      |
      | Program new signal:
      | 6. Reg write tx_enable = 0
      | 7. Go to (1)
  DataIn : Inport
  ValidIn : Inport  Port=2  OutDataTypeStr=boolean
  signal_length : Inport  Port=3  OutDataTypeStr=uint32
  reset : Inport  Port=4  OutDataTypeStr=boolean
  output_enable : Inport  Port=5  OutDataTypeStr=boolean
  Data Type Conversion : DataTypeConversion  OutDataTypeStr=fixdt(0,RAM_addr_width,0)
  Decrement Stored Integer : simulink/Additional Math & Discrete/Additional Math: Increment - Decrement/Decrement Stored Integer
      settings: SourceProductName=Simulink  SourceProductBaseCode=SL
  Detect Rise Positive : simulink/Logic and Bit Operations/Detect Rise Positive  vinit=0  OutDataTypeStr=boolean
  Dual Port RAM : hdlsllib/HDL RAMs/Dual Port RAM  ram_size=RAM_addr_width
      settings: SourceProductName=HDL Coder  SourceProductBaseCode=HD
  Pipeline Delay : Delay  DelayLength=1  InitialCondition=0
  Pipeline Delay1 : Delay  DelayLength=1  InitialCondition=0
  Read Control : MATLAB Function  TreatAsAtomicUnit=on  mask{addr_width=RAM_addr_width}
      mask prompts: addr_width "Address width:"
  Terminator : Terminator
  Unit Delay : UnitDelay  SampleTime=-1  HasFrameUpgradeWarning=on
  Write Control : MATLAB Function  TreatAsAtomicUnit=on  mask{addr_width=RAM_addr_width}
      mask prompts: addr_width "Address width:"
  ZeroOnInvalid : Subsystem
  DataOut : Outport  VectorParamsAs1DForOutWhenUnconnected=off
  ValidOut : Outport  Port=2  VectorParamsAs1DForOutWhenUnconnected=off
  wires:
  ValidIn/1 -> Write Control/2(valid_in)
  Dual Port RAM/1 -> Terminator/1
  signal_length/1 -> Decrement Stored Integer/1
  Data Type Conversion/1 -> Write Control/3(addr_max_in)
  Write Control/2(wr_addr) -> Dual Port RAM/2
  Write Control/3(wr_en) -> Dual Port RAM/3
  Detect Rise Positive/1 -> Write Control/4(reset)
  reset/1 -> Detect Rise Positive/1
  Write Control/1(wr_din) -> Dual Port RAM/1
  DataIn/1 -> Write Control/1(data_in)
  Write Control/4(wr_busy) -> Read Control/1(wr_busy)
  Read Control/1(rd_addr) -> Dual Port RAM/4
  Read Control/2(rd_en) -> Unit Delay/1
  Unit Delay/1 -> ZeroOnInvalid/2(Valid), Pipeline Delay1/1
  output_enable/1 -> Read Control/3(user_enable)
  Write Control/5(addr_max) -> Read Control/2(addr_max)
  Dual Port RAM/2 -> ZeroOnInvalid/1(DataIn)
  Decrement Stored Integer/1 -> Data Type Conversion/1
  ZeroOnInvalid/1(DataOut) -> Pipeline Delay/1
  Pipeline Delay/1 -> DataOut/1
  Pipeline Delay1/1 -> ValidOut/1

== system TxLUT_RxCapture_4x4_HDL_IQ/TxLUT_RxCapture_DUT/Tx LUT/Subsystem/Tx LUT/ZeroOnInvalid ==
  DataIn : Inport
  Valid : Inport  Port=2
  Constant : Constant  Value=0  OutDataTypeStr=Inherit: Inherit via back propagation  SampleTime=-1
  Data Type Duplicate : DataTypeDuplicate
  Multiport Switch : MultiPortSwitch  DataPortOrder=Zero-based contiguous  Inputs=2  zeroidx=on
  DataOut : Outport  VectorParamsAs1DForOutWhenUnconnected=off
  wires:
  Multiport Switch/1 -> DataOut/1
  Constant/1 -> Data Type Duplicate/1, Multiport Switch/2
  Valid/1 -> Multiport Switch/1
  DataIn/1 -> Data Type Duplicate/2, Multiport Switch/3

== matlab function TxLUT_RxCapture_4x4_HDL_IQ/TxLUT_RxCapture_DUT/Tx LUT/Subsystem/Tx LUT/Read Control ==
  data: wr_busy input; addr_max input; user_enable input; rd_addr output; rd_en output; addr_width parameter
function [rd_addr, rd_en] = rd_ctrl(wr_busy, addr_max, user_enable, addr_width)

persistent addr_next user_enable_prev

if isempty(addr_next)
    addr_next = fi(0, 0,addr_width,0);
    user_enable_prev = false;
end

%% Assign register values to signals
addr = addr_next;

%% Internal signals
enabled = user_enable && ~wr_busy;
reset = user_enable && ~user_enable_prev;

%% Update registers
if enabled
    if addr >= addr_max
        addr_next(:) = 0;
    else
        addr_next(:) = addr + 1;
    end
end

if reset
    addr_next(:) = 0;
end

user_enable_prev = user_enable;
    
%% Outputs
rd_addr = addr;
rd_en = enabled;

== matlab function TxLUT_RxCapture_4x4_HDL_IQ/TxLUT_RxCapture_DUT/Tx LUT/Subsystem/Tx LUT/Write Control ==
  data: data_in input; wr_din output; valid_in input; wr_addr output; addr_max_in input; reset input; wr_en output; addr_width parameter; wr_busy output; addr_max output
function [wr_din, wr_addr, wr_en, wr_busy, addr_max] = ...
    wr_ctrl(data_in, valid_in, addr_max_in, reset, addr_width)

STATE_IDLE  = coder.const(fi(0, 0,2,0));
STATE_WRITE = coder.const(fi(1, 0,2,0));
STATE_WAIT  = coder.const(fi(2, 0,2,0));

persistent state_next data_next valid_next addr_next addr_max_next

if isempty(state_next)
    state_next = STATE_IDLE;
    data_next = zeros(1,1,'like',data_in);
    valid_next = false;
    addr_next = fi(0, 0,addr_width,0);
    addr_max_next = fi(2^addr_width - 1, 0,addr_width,0);
end

%% Assign register values to signals
state = state_next;
data = data_next;
valid = valid_next;
addr = addr_next;
addr_max = addr_max_next;

%% State transition logic
en = false;
switch state
    
    % Idle
    case STATE_IDLE
        
        if valid_in
            state_next = STATE_WRITE;
            addr_max_next(:) = addr_max_in;
            addr_next(:) = 0;
        end
        
    % Writing to RAM
    case STATE_WRITE
        
        if reset
            state_next = STATE_IDLE;
        elseif (addr == addr_max) && valid
            state_next = STATE_WAIT;
        end
        
        if valid
           addr_next(:) = addr + 1;
           en = true;
        end
        
    % Waiting for reset signal
    case STATE_WAIT
        
        if reset
            state_next = STATE_IDLE;
        end
        
    otherwise
        state_next = STATE_IDLE;
end

%% Update data/valid registers
data_next = data_in;
valid_next = valid_in;
    
%% Outputs
wr_din = data;
wr_addr = addr;
wr_en = en;
wr_busy = (state == STATE_WRITE);
